simulink model "curva_modulo"  (R2021a)
settings: Solver=ode23t  StartTime=0.0  StopTime=20  MaxStep=1e-6  RelTol=1e-3
values from neighbouring files (symbols this model uses):
  Ir = 1000    [curva_excel.m]
  T = 25*j    [curva_excel.m]
  Voc = str2num(get_param('curva_modulo/PV Array','Voc'))    [curva_excel.m]
libraries: spsControlledVoltageSourceLib x1, spsCurrentMeasurementLib x1, spsPVArrayLib x1, simulink x1, spsVoltageMeasurementLib x1, spspowerguiLib x1
settings Model: Creator=junio  LastModifiedBy=junio

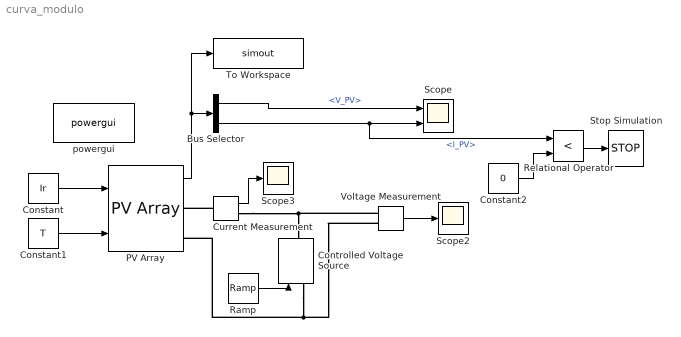
== system curva_modulo ==
  Bus Selector : BusSelector  OutputSignals=V_PV,I_PV
  Constant : Constant  Value=Ir
  Constant1 : Constant  Value=T
  Constant2 : Constant  Value=0
  Controlled Voltage Source : spsControlledVoltageSourceLib/Controlled Voltage Source  Initialize=on  Source_Type=DC  Amplitude=0  Phase=0  Frequency=0  Measurements=None
  Current Measurement : spsCurrentMeasurementLib/Current Measurement  PhasorSimulation=off  OutputType=Complex  PSBequivalent=0
  PV Array : spsPVArrayLib/PV Array  Npar=1  Nser=1  PlotType=array @ 1000 W/m2 & specified temperatures  S_vec="[ 1000  500  100 ]"  Temp_C_vec="[ 45 25  ]"  ModuleName=Advance Power API-M230  PlotWhenSelected=off  Pm=230.124  Ncell=60  Voc=37.32  Isc=8.18  Vm=30.48  Im=7.55  beta_Voc_pc=-0.3564  alpha_Isc_pc=0.053729  beta_Voc=-0.13301  alpha_Isc=0.004395  IL=8.1984  I0=2.4009e-10  nI=0.99962  Rsh=131.8863  Rs=0.29686  RobustModel=off  RobustCellTemperature=313.3991  BAL=on  Tc=1e-6  Tfilter=5e-5
  Ramp : simulink/Sources/Ramp  slope=Voc  start=0  InitialOutput=0
  Relational Operator : RelationalOperator  Operator=<  OutDataTypeStr=boolean  RndMeth=Simplest
  Scope : Scope  NumInputPorts=2
  Scope2 : Scope
  Scope3 : Scope
  Stop Simulation : Stop
  To Workspace : ToWorkspace  VariableName=simout  SaveFormat=Timeseries  SampleTime=-1
  Voltage Measurement : spsVoltageMeasurementLib/Voltage Measurement  PhasorSimulation=off  OutputType=Complex  PSBequivalent=0
  powergui : spspowerguiLib/powergui  Priority=1  SimulationMode=Continuous  SampleTime=50e-6  frequency=60  Iterations=50  frequencyindice=0  Pbase=100e6  ErrMax=1e-4  UnitsV=kV  UnitsW=MW  buscounter=0  FunctionMessages=off  echomessages=off  EnableUseOfTLC=off  CurrentSourceSwitches=off  DisableSnubberDevices=off  DisableRonSwitches=off  DisableVfSwitches=off  DisplayEquations=off  AutomaticDiscreteSolvers=off  SolverType=Tustin/Backward Euler (TBE)  Interpol=off  ExternalGateDelay=off  methode=off  Ts=100  x0status=blocks  SPID=on  SwTol=0  HookPort=off  NonlinearTolerance=1e-4  nMaxIteration=100  ContinueOnMaxIteration=off  RestoreLinks=warning  ResistiveCurrentMeasurement=off  Frange=[0:2:500]  Ylog=off  Xlog=on  ShowGrid=off  save=off  variable=ZData  structure=0  ZoomFFT=off  StartTime=0.0  cycles=1  DisplayStyle=1  fundamental=60  FreqAxis=off  MaxFrequency=1000  frequencyindicesteady=1  RmsSteady=1  display=off
  wires:
  Constant/1 -> PV Array/1
  Constant1/1 -> PV Array/2
  PV Array/1 -> To Workspace/1, Bus Selector/1
  Bus Selector/2 -> Scope/2, Relational Operator/1  "<I_PV>"
  Bus Selector/1 -> Scope/1  "<V_PV>"
  Ramp/1 -> Controlled Voltage Source/1
  Voltage Measurement/1 -> Scope2/1
  Current Measurement/1 -> Scope3/1
  Constant2/1 -> Relational Operator/2
  Relational Operator/1 -> Stop Simulation/1
  connections:
  Current Measurement/LConn1 -- PV Array/RConn1
  Voltage Measurement/LConn2 -- Controlled Voltage Source/LConn1 -- PV Array/RConn2
  Current Measurement/RConn1 -- Voltage Measurement/LConn1 -- Controlled Voltage Source/RConn1
